simulink model "FOC_Control_doubleLoop"  (R2023a)
settings: Solver=FixedStepDiscrete  StartTime=0.0  StopTime=5  FixedStep=0.000001  RelTol=1e-3  EnableMultiTasking=on
InitFcn:
  | SPEED_PI_P=0.03
  | SPEED_PI_I=5
  | SPEED_PI_UP_LIMIT = 5.0
  | SPEED_PI_LOW_LIMIT = -5.0
  | SPEED_PI_KB = 0.015
  | D_PI_P = 2.199
  | D_PI_I = 1282.8
  | D_PI_UP_LIMIT = 24.0
  | D_PI_LOW_LIMIT = -24.0
  | D_PI_KB = 15
  | Q_PI_P = 2.199
  | Q_PI_I = 1282.8
  | Q_PI_UP_LIMIT = 24.0
  | Q_PI_LOW_LIMIT = -24.0
  | Q_PI_KB = 15
libraries: slpidlib x3, spsDCVoltageSourceLib x1, spsGroundLib x1, spsPermanentMagnetSynchronousMachineLib x1, simulink x1, spsThreePhaseVIMeasurementLib x1, spsUniversalBridgeLib x1, spspowerguiLib x1
settings Model: ExtModeTrigDuration=5  TunableVars=D_PI_I,D_PI_KB,D_PI_LIMIT,D_PI_LOW_LIMIT,D_PI_P,D_PI_UP_LIMIT,Q_PI_I,Q_PI_KB,Q_PI_LIMIT,Q_PI_LOW_LIMIT,Q_PI_P,Q_PI_UP_LIMIT,SPEED_PI_I,SPEED_PI_KB,SPEED_PI_LIMIT,SPEED_PI_LOW_LIMIT,SPEED_PI_P,SPEED_PI_UP_LIMIT  TunableVarsStorageClass=Auto,Auto,Auto,Auto,Auto,Auto,Auto,Auto,Auto,Auto,Auto,Auto,Auto,Auto,Auto,Auto,Auto,Auto  TunableVarsTypeQualifier=,,,,,,,,,,,,,,,,,  Creator=wang  LastModifiedBy=28076
settings SolverCC: AlgebraicLoopSolver=TrustRegion
settings DataIOCC: ReturnWorkspaceOutputs=off
settings OptimizationCC: DefaultParameterBehavior=Inlined  UseDivisionForNetSlopeComputation=on  GainParamInheritBuiltInType=on  UseFloatMulNetSlope=on  DefaultUnderspecifiedDataType=single  InlineInvariantSignals=on  PassReuseOutputArgsAs=Individual arguments  ZeroExternalMemoryAtStartup=off  ZeroInternalMemoryAtStartup=off  NoFixptDivByZeroProtection=on  EfficientFloat2IntCast=on  LifeSpan=1  MaxStackSize=64  OptimizeBlockOrder=speed  DifferentSizesBufferReuse=on  EfficientTunableParamExpr=on
settings DebuggingCC: ParameterTunabilityLossMsg=error  UnconnectedInputMsg=warning  UnconnectedOutputMsg=warning  UnconnectedLineMsg=warning  ArithmeticOperatorsInVariantConditions=warning
settings HardwareCC: ProdBitPerPointer=32  ProdBitPerSizeT=32  ProdBitPerPtrDiffT=32  ProdLargestAtomicInteger=Long  ProdLargestAtomicFloat=Double  ProdWordSize=32  ProdLongLongMode=on  ProdHWDeviceType=ARM Compatible->ARM Cortex
settings ModelReferenceCC: EnableRefExpFcnMdlSchedulingChecks=on
settings SFSimCC: MATLABDynamicMemAlloc=off  CustomCodeUndefinedFunction=UseInterfaceOnly
settings RTWCC: Description=Embedded Coder  SystemTargetFile=ert.tlc  HardwareBoard=NXP FRDM-K64F  TLCOptions="-aInlineSetEventsForThisBaseRateFcn=TLC_FALSE -aSuppressMultiTaskScheduler=TLC_FALSE    -aRateBasedStepFcn=0"  TemplateMakefile=ert_default_tmf  GenerateReport=on  Toolchain=GNU Tools for ARM Embedded Processors  IncludeHyperlinkInReport=on  LaunchReport=on  GenerateTraceInfo=on  GenerateTraceReport=on  GenerateTraceReportSl=on  GenerateTraceReportSf=on  GenerateTraceReportEml=on  GenerateCodeMetricsReport=on  DLArmComputeVersion=19.05
settings CodeAppCC: ForceParamTrailComments=on  IgnoreCustomStorageClasses=off  OperatorAnnotations=on  SimulinkDataObjDesc=on  SFDataObjDesc=on  CustomSymbolStrGlobalVar=rt$N$M  CustomSymbolStrType=$N$M  CustomSymbolStrFcn=$N$M$F  CustomSymbolStrMacro=$N$M  InsertBlockDesc=on
settings ERTTargetCC: CodeReplacementLibrary=ARM Cortex-M (Optimized)  IncludeMdlTerminateFcn=off  CombineSignalStateStructs=on  SupportComplex=off  SupportNonInlinedSFcns=on  ExtModeTransport=4  ExtModeMexFile=sendToCommService  InlinedParameterPlacement=NonHierarchical  ERTSrcFileBannerTemplate=mbd_s32k3_ert_code_template.cgt  ERTHdrFileBannerTemplate=mbd_s32k3_ert_code_template.cgt  ERTDataSrcFileTemplate=mbd_s32k3_ert_code_template.cgt  ERTDataHdrFileTemplate=mbd_s32k3_ert_code_template.cgt  ERTFilePackagingFormat=CompactWithDataFile
settings ConfigComp: PSAutoStubLUT=on

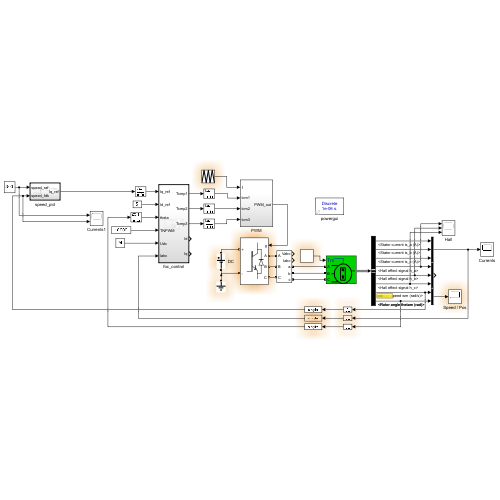
[thumbnail: Simulink's stored preview of the top-level diagram]
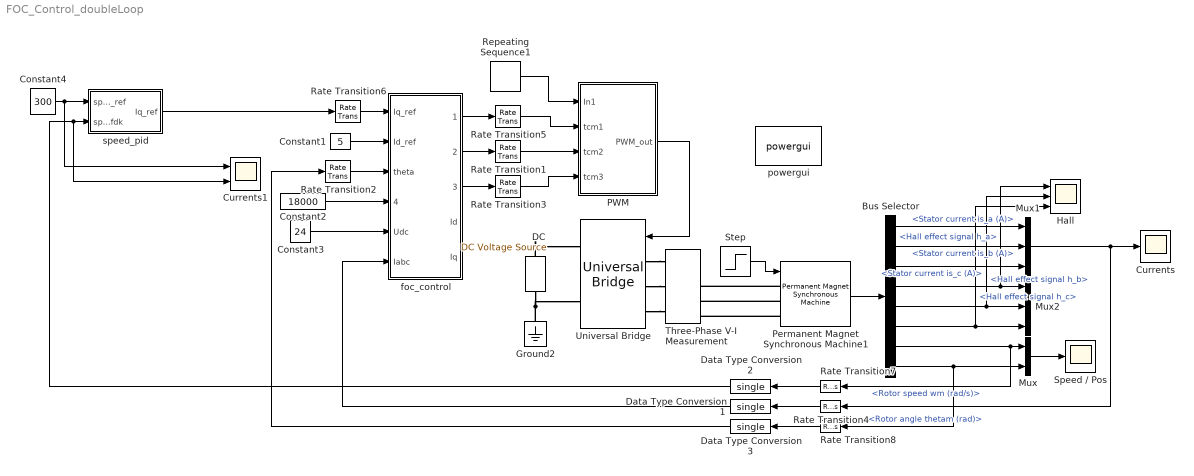
== system FOC_Control_doubleLoop ==
  Bus Selector : BusSelector  OutputSignals=Stator current is_a (A),Stator current is_b (A),Stator current is_c (A),Hall effect signal h_a,Hall effect signal h_b,Hall effect signal h_c,Rotor speed wm (rad/s),Rotor angle thetam (rad)
  Constant1 : Constant  Value=5  OutDataTypeStr=single
  Constant2 : Constant  Value=18000  OutDataTypeStr=single
  Constant3 : Constant  Value=24  OutDataTypeStr=single
  Constant4 : Constant  Value=300  OutDataTypeStr=single
  Currents : Scope
  Currents1 : Scope  NumInputPorts=2
  "DC " : spsDCVoltageSourceLib/DC Voltage Source  Amplitude=24  Measurements=None
  Data Type Conversion1 : DataTypeConversion  OutDataTypeStr=single  SaturateOnIntegerOverflow=off  RndMeth=Floor
  Data Type Conversion2 : DataTypeConversion  OutDataTypeStr=single  SaturateOnIntegerOverflow=off  RndMeth=Floor
  Data Type Conversion3 : DataTypeConversion  OutDataTypeStr=single  SaturateOnIntegerOverflow=off  RndMeth=Floor
  Ground2 : spsGroundLib/Ground  LConnTagsString=a
  Hall : Scope  NumInputPorts=3
  Mux : Mux  Inputs=2
  Mux1 : Mux  Inputs=3
  Mux2 : Mux  Inputs=3
  PWM : Subsystem
  Permanent Magnet Synchronous Machine1 : spsPermanentMagnetSynchronousMachineLib/Permanent Magnet Synchronous Machine  NbPhases=3  FluxDistribution=Sinusoidal  RotorType=Round  MechanicalLoad=Torque Tm  PresetModel=No  ShowDetailedParameters=on  MeasurementBus=off  Resistance=0.6  Inductance=8.5e-3  dqInductances=[8.5e-3, 8.5e-3]  La=1.4e-3  MachineConstant=Flux linkage established by magnets (V.s)  Flux=0.034182  VoltageCst=6.1999  TorqueCst=0.051273  Flat=120  Mechanical=[1.1e-5,1e-4,1,0.02]  PolePairs=4  InitialConditions=[0,0, 0,0]  InitialConditions5ph=[0 0 0 0 0 0]  RefAngle=Aligned with phase A axis (original Park)  IterativeDiscreteModel=Trapezoidal non iterative  TsBlock=-1  TsPowergui=0
  Rate Transition{1..8} (8 alike) : RateTransition
  Repeating Sequence1 : simulink/Sources/Repeating Sequence  rep_seq_t=[0 0.0001 0.0002]  rep_seq_y=[0 9000 0]
  Speed / Pos : Scope
  Step : Step  Time=0  After=0  SampleTime=0
  Three-Phase V-I Measurement : spsThreePhaseVIMeasurementLib/Three-Phase V-I Measurement  VoltageMeasurement=phase-to-ground  SetLabelV=off  LabelV=Vabc  Vpu=off  VpuLL=off  CurrentMeasurement=yes  SetLabelI=off  LabelI=Iabc  Ipu=off  Pbase=100e6  Vbase=500e3  OutputType=Complex  PhasorSimulation=off  PSBequivalent=0
  Universal Bridge : spsUniversalBridgeLib/Universal Bridge  Arms=3  SnubberResistance=1e5  SnubberCapacitance=inf  Device=IGBT / Diodes  Ron=1e-3  Lon=0  ForwardVoltages="[  0  0  ]"  ForwardVoltage=0  GTOparameters=[ 10e-6 , 20e-6 ]  IGBTparameters=[ 1e-6 , 2e-6 ]  Measurements=None  Measurements_2=None  converterType=Rectifier
  foc_control : Subsystem  TreatAsAtomicUnit=on  SystemSampleTime=0.0001
  powergui : spspowerguiLib/powergui  Priority=1  SimulationMode=Discrete  SampleTime=0.000001  frequency=60  Iterations=50  frequencyindice=0  Pbase=100e6  ErrMax=1e-4  UnitsV=kV  UnitsW=MW  buscounter=0  FunctionMessages=off  echomessages=off  EnableUseOfTLC=off  CurrentSourceSwitches=off  DisableSnubberDevices=off  DisableRonSwitches=off  DisableVfSwitches=off  DisplayEquations=off  AutomaticDiscreteSolvers=off  SolverType=Tustin/Backward Euler (TBE)  Interpol=off  ExternalGateDelay=off  methode=off  Ts=100  x0status=blocks  SPID=off  SwTol=0  HookPort=off  NonlinearTolerance=1e-4  nMaxIteration=100  ContinueOnMaxIteration=off  RestoreLinks=warning  ResistiveCurrentMeasurement=off  Frange=[0:2:500]  Ylog=off  Xlog=on  ShowGrid=off  save=off  variable=ZData  structure=0  ZoomFFT=off  StartTime=0.0  cycles=1  DisplayStyle=1  fundamental=60  FreqAxis=off  MaxFrequency=1000  frequencyindicesteady=1  RmsSteady=1  display=off
  speed_pid : Subsystem  TreatAsAtomicUnit=on  SystemSampleTime=0.001
  wires:
  Constant1/1 -> foc_control/2(Id_ref)
  Constant2/1 -> foc_control/4(TNPWM)
  Constant3/1 -> foc_control/5(Udc)
  Repeating Sequence1/1 -> PWM/1(In1)
  foc_control/1(Tcmp1) -> Rate Transition5/1
  foc_control/2(Tcmp2) -> Rate Transition1/1
  foc_control/3(Tcmp3) -> Rate Transition3/1
  PWM/1(PWM_out) -> Universal Bridge/1
  Bus Selector/4 -> Hall/1, Mux2/1  "<Hall effect signal h_a>"
  Mux/1 -> Speed / Pos/1
  Bus Selector/2 -> Mux1/2  "<Stator current is_b (A)>"
  Bus Selector/7 -> Rate Transition7/1, Mux/1  "<Rotor speed wm (rad/s)>"
  Bus Selector/5 -> Mux2/2, Hall/2  "<Hall effect signal h_b>"
  Bus Selector/6 -> Mux2/3, Hall/3  "<Hall effect signal h_c>"
  Mux1/1 -> Rate Transition4/1, Currents/1
  Bus Selector/1 -> Mux1/1  "<Stator current is_a (A)>"
  Bus Selector/8 -> Rate Transition8/1, Mux/2  "<Rotor angle thetam (rad)>"
  Bus Selector/3 -> Mux1/3  "<Stator current is_c (A)>"
  Permanent Magnet Synchronous Machine1/1 -> Bus Selector/1
  Rate Transition2/1 -> foc_control/3(theta)
  Rate Transition5/1 -> PWM/2(tcm1)
  Rate Transition1/1 -> PWM/3(tcm2)
  Rate Transition3/1 -> PWM/4(tcm3)
  Step/1 -> Permanent Magnet Synchronous Machine1/1
  Rate Transition4/1 -> Data Type Conversion1/1
  Data Type Conversion1/1 -> foc_control/6(Iabc)
  Constant4/1 -> Currents1/1, speed_pid/1(speed_ref)
  Rate Transition6/1 -> foc_control/1(Iq_ref)
  Rate Transition7/1 -> Data Type Conversion2/1
  Rate Transition8/1 -> Data Type Conversion3/1
  Data Type Conversion2/1 -> Currents1/2, speed_pid/2(speed_fdk)
  Data Type Conversion3/1 -> Rate Transition2/1
  speed_pid/1(Iq_ref) -> Rate Transition6/1
  connections:
  Ground2/LConn1 -- Universal Bridge/RConn2 -- "DC "/LConn1
  Universal Bridge/LConn1 -- Three-Phase V-I Measurement/LConn1
  Universal Bridge/LConn2 -- Three-Phase V-I Measurement/LConn2
  "DC "/RConn1 -- Universal Bridge/RConn1
  Universal Bridge/LConn3 -- Three-Phase V-I Measurement/LConn3
  Permanent Magnet Synchronous Machine1/LConn1 -- Three-Phase V-I Measurement/RConn1
  Permanent Magnet Synchronous Machine1/LConn2 -- Three-Phase V-I Measurement/RConn2
  Permanent Magnet Synchronous Machine1/LConn3 -- Three-Phase V-I Measurement/RConn3

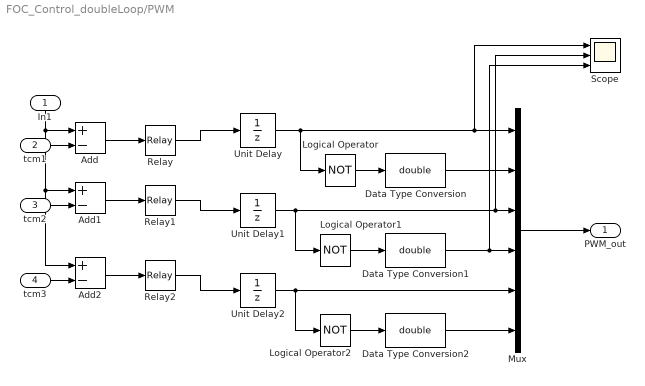
== system FOC_Control_doubleLoop/PWM ==
  In1 : Inport
  tcm1 : Inport  Port=2
  tcm2 : Inport  Port=3
  tcm3 : Inport  Port=4
  Add : Sum  Inputs=+-
  Add1 : Sum  Inputs=+-
  Add2 : Sum  Inputs=+-
  Data Type Conversion : DataTypeConversion  OutDataTypeStr=double  SaturateOnIntegerOverflow=off  RndMeth=Floor
  Data Type Conversion1 : DataTypeConversion  OutDataTypeStr=double  SaturateOnIntegerOverflow=off  RndMeth=Floor
  Data Type Conversion2 : DataTypeConversion  OutDataTypeStr=double  SaturateOnIntegerOverflow=off  RndMeth=Floor
  Logical Operator : Logic  Operator=NOT  AllPortsSameDT=off  OutDataTypeStr=boolean
  Logical Operator1 : Logic  Operator=NOT  AllPortsSameDT=off  OutDataTypeStr=boolean
  Logical Operator2 : Logic  Operator=NOT  AllPortsSameDT=off  OutDataTypeStr=boolean
  Mux : Mux  Inputs=6
  Relay : Relay  OffSwitchValue=-eps
  Relay1 : Relay  OffSwitchValue=-eps
  Relay2 : Relay  OffSwitchValue=-eps
  Scope : Scope  NumInputPorts=3
  Unit Delay : UnitDelay  SampleTime=-1  HasFrameUpgradeWarning=on
  Unit Delay1 : UnitDelay  SampleTime=-1  HasFrameUpgradeWarning=on
  Unit Delay2 : UnitDelay  SampleTime=-1  HasFrameUpgradeWarning=on
  PWM_out : Outport  VectorParamsAs1DForOutWhenUnconnected=off
  wires:
  tcm3/1 -> Add2/2
  tcm2/1 -> Add1/2
  tcm1/1 -> Add/2
  Relay2/1 -> Unit Delay2/1
  Relay1/1 -> Unit Delay1/1
  Relay/1 -> Unit Delay/1
  Unit Delay2/1 -> Mux/5, Logical Operator2/1
  Unit Delay1/1 -> Scope/2, Mux/3, Logical Operator1/1
  Unit Delay/1 -> Logical Operator/1, Scope/1, Mux/1
  Mux/1 -> PWM_out/1
  Data Type Conversion/1 -> Mux/2
  Data Type Conversion1/1 -> Scope/3, Mux/4
  Data Type Conversion2/1 -> Mux/6
  Logical Operator2/1 -> Data Type Conversion2/1
  Logical Operator1/1 -> Data Type Conversion1/1
  Logical Operator/1 -> Data Type Conversion/1
  Add1/1 -> Relay1/1
  Add2/1 -> Relay2/1
  Add/1 -> Relay/1
  In1/1 -> Add/1, Add2/1, Add1/1

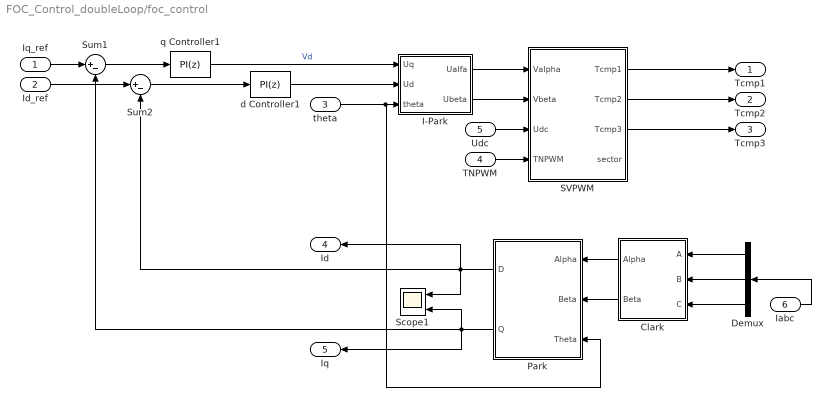
== system FOC_Control_doubleLoop/foc_control ==
  Iq_ref : Inport  OutDataTypeStr=single
  Id_ref : Inport  Port=2  OutDataTypeStr=single
  theta : Inport  Port=3  OutDataTypeStr=single
  TNPWM : Inport  Port=4  OutDataTypeStr=single
  Udc : Inport  Port=5  OutDataTypeStr=single
  Iabc : Inport  Port=6  OutDataTypeStr=single
  Clark : Subsystem
  Demux : Demux  Outputs=3
  I-Park : Subsystem
  Park : Subsystem
  SVPWM : MATLAB Function  TreatAsAtomicUnit=on
  Scope1 : Scope  NumInputPorts=2
  Sum1 : Sum  Inputs=|+-
  Sum2 : Sum  Inputs=|+-
  d Controller1 : slpidlib/PID Controller  Controller=PI  Form=Parallel  TimeDomain=Discrete-time  UseExternalTs=off  SampleTime=-1  IntegratorMethod=Forward Euler  FilterMethod=Forward Euler  ControllerParametersSource=internal  P=D_PI_P  I=D_PI_I  UseKiTs=off  D=0.09  N=100  UseFilter=on  TunerSelectOption=Transfer Function Based (PID Tuner App)  InitialConditionSource=internal  InitialConditionForIntegrator=0  InitialConditionForFilter=0  DifferentiatorICPrevScaledInput=0  ExternalReset=none  TrackingMode=off  Kt=1  LimitOutput=on  SatLimitsSource=internal  UpperSaturationLimit=D_PI_UP_LIMIT  LowerSaturationLimit=D_PI_LOW_LIMIT  LinearizeAsGain=off  AntiWindupMode=back-calculation  Kb=D_PI_KB  LimitIntegrator=off  UpperIntegratorSaturationLimit=inf  LowerIntegratorSaturationLimit=-inf  PGainOutDataTypeStr=single  PProdOutDataTypeStr=single  POutMin=[]  POutMax=[]  IGainOutDataTypeStr=single  IProdOutDataTypeStr=single  IOutMin=[]  IOutMax=[]  DOutMin=[]  DOutMax=[]  NOutMin=[]  NOutMax=[]  SumOutDataTypeStr=single  SumOutMin=[]  SumOutMax=[]  SaturationOutDataTypeStr=single  SaturationOutMin=[]  SaturationOutMax=[]  PParamDataTypeStr=single  PParamMin=[]  PParamMax=[]  IParamDataTypeStr=single  IParamMin=[]  IParamMax=[]  DParamMin=[]  DParamMax=[]  NParamMin=[]  NParamMax=[]  KbParamDataTypeStr=single  KbParamMin=[]  KbParamMax=[]  KtParamMin=[]  KtParamMax=[]  KbOutDataTypeStr=single  KbOutMin=[]  KbOutMax=[]  KtOutMin=[]  KtOutMax=[]  IntegratorOutDataTypeStr=single  IntegratorOutMin=[]  IntegratorOutMax=[]  FilterOutMin=[]  FilterOutMax=[]  SumI1OutDataTypeStr=single  SumI1OutMin=[]  SumI1OutMax=[]  SumI2OutDataTypeStr=single  SumI2OutMin=[]  SumI2OutMax=[]  SumI3OutMin=[]  SumI3OutMax=[]  SumI4OutMin=[]  SumI4OutMax=[]  SumDOutMin=[]  SumDOutMax=[]  SumAccumDataTypeStr=single  SumI1AccumDataTypeStr=single  SumI2AccumDataTypeStr=single  DifferentiatorOutMin=[]  DifferentiatorOutMax=[]  FilterDiffOutCoefMin=[]  FilterDiffOutCoefMax=[]  ReciprocalOutMin=[]  ReciprocalOutMax=[]  SumDenOutMin=[]  SumDenOutMax=[]  SumNumOutMin=[]  SumNumOutMax=[]  DivideOutMin=[]  DivideOutMax=[]  UdiffTsProdOutMin=[]  UdiffTsProdOutMax=[]  NTsProdOutMin=[]  NTsProdOutMax=[]  UintegralTsProdOutMin=[]  UintegralTsProdOutMax=[]  UngainTsProdOutMin=[]  UngainTsProdOutMax=[]  ClampingZeroOutDataTypeStr=Inherit: Inherit via back propagation  ClampingZeroOutMin=[]  ClampingZeroOutMax=[]  FilterDenConstantOutDataTypeStr=Inherit: Inherit via back propagation  FilterDenConstantOutMin=[]  FilterDenConstantOutMax=[]  PCopyOutDataTypeStr=Inherit: Inherit via back propagation  PCopyOutMin=[]  PCopyOutMax=[]  NCopyOutDataTypeStr=Inherit: Inherit via back propagation  NCopyOutMin=[]  NCopyOutMax=[]  IntegratorContinuousStateAttributes=''  IntegratorStateIdentifier=di  IntegratorStateMustResolveToSignalObject=off  IntegratorRTWStateStorageClass=Auto  FilterContinuousStateAttributes=''  FilterStateMustResolveToSignalObject=off  FilterRTWStateStorageClass=Auto  ParallelPVariant=InternalParameters  IdealPVariant=Disabled  IVariant=InternalParameters  DVariant=Disabled  IntegratorVariant=Discrete  SatVariant=Enabled  AWVariant=BackCalculation  PCopyVariant=Disabled  TRVariant=Disabled  FdbkBlocksVariant=Forward  IdealPFdbkVariant=Disabled  SatFdbkVariant=Disabled  DerivativeFilterVariant=Disabled  NVariant=Disabled  NCopyVariant=Disabled_SignalSpec  FilterICVariant=Disabled  IntegratorICVariant=InternalICs  ExternalResetVariant=Disabled  TRSumVariant=Passthrough  SumFdbkVariant=Disabled  SumVariant=Sum_PI  TsampFilterVariant=InternalTs  TsampNgainVariant=Passthrough  TsampIntegralVariant=Disabled_SignalSpec  ExternalSaturationOutDataTypeStr=Inherit: Same as second input
  q Controller1 : slpidlib/PID Controller  Controller=PI  Form=Parallel  TimeDomain=Discrete-time  UseExternalTs=off  SampleTime=-1  IntegratorMethod=Forward Euler  FilterMethod=Forward Euler  ControllerParametersSource=internal  P=Q_PI_P  I=Q_PI_I  UseKiTs=off  D=0.09  N=100  UseFilter=on  TunerSelectOption=Transfer Function Based (PID Tuner App)  InitialConditionSource=internal  InitialConditionForIntegrator=0  InitialConditionForFilter=0  DifferentiatorICPrevScaledInput=0  ExternalReset=none  TrackingMode=off  Kt=1  LimitOutput=on  SatLimitsSource=internal  UpperSaturationLimit=Q_PI_UP_LIMIT  LowerSaturationLimit=Q_PI_LOW_LIMIT  LinearizeAsGain=off  AntiWindupMode=back-calculation  Kb=Q_PI_KB  LimitIntegrator=off  UpperIntegratorSaturationLimit=inf  LowerIntegratorSaturationLimit=-inf  PGainOutDataTypeStr=single  PProdOutDataTypeStr=single  POutMin=[]  POutMax=[]  IGainOutDataTypeStr=single  IProdOutDataTypeStr=single  IOutMin=[]  IOutMax=[]  DOutMin=[]  DOutMax=[]  NOutMin=[]  NOutMax=[]  SumOutDataTypeStr=single  SumOutMin=[]  SumOutMax=[]  SaturationOutDataTypeStr=single  SaturationOutMin=[]  SaturationOutMax=[]  PParamDataTypeStr=single  PParamMin=[]  PParamMax=[]  IParamDataTypeStr=single  IParamMin=[]  IParamMax=[]  DParamMin=[]  DParamMax=[]  NParamMin=[]  NParamMax=[]  KbParamDataTypeStr=single  KbParamMin=[]  KbParamMax=[]  KtParamMin=[]  KtParamMax=[]  KbOutDataTypeStr=single  KbOutMin=[]  KbOutMax=[]  KtOutMin=[]  KtOutMax=[]  IntegratorOutDataTypeStr=single  IntegratorOutMin=[]  IntegratorOutMax=[]  FilterOutMin=[]  FilterOutMax=[]  SumI1OutDataTypeStr=single  SumI1OutMin=[]  SumI1OutMax=[]  SumI2OutDataTypeStr=single  SumI2OutMin=[]  SumI2OutMax=[]  SumI3OutMin=[]  SumI3OutMax=[]  SumI4OutMin=[]  SumI4OutMax=[]  SumDOutMin=[]  SumDOutMax=[]  SumAccumDataTypeStr=single  SumI1AccumDataTypeStr=single  SumI2AccumDataTypeStr=single  DifferentiatorOutMin=[]  DifferentiatorOutMax=[]  FilterDiffOutCoefMin=[]  FilterDiffOutCoefMax=[]  ReciprocalOutMin=[]  ReciprocalOutMax=[]  SumDenOutMin=[]  SumDenOutMax=[]  SumNumOutMin=[]  SumNumOutMax=[]  DivideOutMin=[]  DivideOutMax=[]  UdiffTsProdOutMin=[]  UdiffTsProdOutMax=[]  NTsProdOutMin=[]  NTsProdOutMax=[]  UintegralTsProdOutMin=[]  UintegralTsProdOutMax=[]  UngainTsProdOutMin=[]  UngainTsProdOutMax=[]  ClampingZeroOutDataTypeStr=Inherit: Inherit via back propagation  ClampingZeroOutMin=[]  ClampingZeroOutMax=[]  FilterDenConstantOutDataTypeStr=Inherit: Inherit via back propagation  FilterDenConstantOutMin=[]  FilterDenConstantOutMax=[]  PCopyOutDataTypeStr=Inherit: Inherit via back propagation  PCopyOutMin=[]  PCopyOutMax=[]  NCopyOutDataTypeStr=Inherit: Inherit via back propagation  NCopyOutMin=[]  NCopyOutMax=[]  IntegratorContinuousStateAttributes=''  IntegratorStateIdentifier=qi  IntegratorStateMustResolveToSignalObject=off  IntegratorRTWStateStorageClass=Auto  FilterContinuousStateAttributes=''  FilterStateMustResolveToSignalObject=off  FilterRTWStateStorageClass=Auto  ParallelPVariant=InternalParameters  IdealPVariant=Disabled  IVariant=InternalParameters  DVariant=Disabled  IntegratorVariant=Discrete  SatVariant=Enabled  AWVariant=BackCalculation  PCopyVariant=Disabled  TRVariant=Disabled  FdbkBlocksVariant=Forward  IdealPFdbkVariant=Disabled  SatFdbkVariant=Disabled  DerivativeFilterVariant=Disabled  NVariant=Disabled  NCopyVariant=Disabled_SignalSpec  FilterICVariant=Disabled  IntegratorICVariant=InternalICs  ExternalResetVariant=Disabled  TRSumVariant=Passthrough  SumFdbkVariant=Disabled  SumVariant=Sum_PI  TsampFilterVariant=InternalTs  TsampNgainVariant=Passthrough  TsampIntegralVariant=Disabled_SignalSpec  ExternalSaturationOutDataTypeStr=Inherit: Same as second input
  Tcmp1 : Outport  VectorParamsAs1DForOutWhenUnconnected=off
  Tcmp2 : Outport  Port=2  VectorParamsAs1DForOutWhenUnconnected=off
  Tcmp3 : Outport  Port=3  VectorParamsAs1DForOutWhenUnconnected=off
  Id : Outport  Port=4  VectorParamsAs1DForOutWhenUnconnected=off
  Iq : Outport  Port=5  VectorParamsAs1DForOutWhenUnconnected=off
  wires:
  I-Park/1(Ualfa) -> SVPWM/1(Valpha)
  theta/1 -> Park/3(Theta), I-Park/3(theta)
  I-Park/2(Ubeta) -> SVPWM/2(Vbeta)
  d Controller1/1 -> I-Park/2(Ud)
  Udc/1 -> SVPWM/3(Udc)
  TNPWM/1 -> SVPWM/4(TNPWM)
  SVPWM/1(Tcmp1) -> Tcmp1/1
  SVPWM/2(Tcmp2) -> Tcmp2/1
  SVPWM/3(Tcmp3) -> Tcmp3/1
  Clark/1(Alpha) -> Park/1(Alpha)
  Clark/2(Beta) -> Park/2(Beta)
  Demux/3 -> Clark/3(C)
  Iabc/1 -> Demux/1
  Park/1(D) -> Sum2/2, Id/1, Scope1/1
  Park/2(Q) -> Sum1/2, Iq/1, Scope1/2
  Demux/2 -> Clark/2(B)
  Demux/1 -> Clark/1(A)
  Sum1/1 -> q Controller1/1
  Sum2/1 -> d Controller1/1
  Iq_ref/1 -> Sum1/1
  Id_ref/1 -> Sum2/1
  q Controller1/1 -> I-Park/1(Uq)  "Vd"

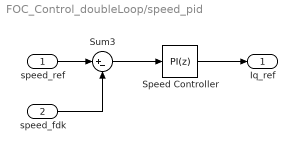
== system FOC_Control_doubleLoop/speed_pid ==
  speed_ref : Inport
  speed_fdk : Inport  Port=2
  Speed Controller : slpidlib/PID Controller  Controller=PI  Form=Ideal  TimeDomain=Discrete-time  UseExternalTs=off  SampleTime=-1  IntegratorMethod=Forward Euler  FilterMethod=Forward Euler  ControllerParametersSource=internal  P=SPEED_PI_P  I=SPEED_PI_I  UseKiTs=off  D=0.0005  N=100  UseFilter=on  TunerSelectOption=Transfer Function Based (PID Tuner App)  InitialConditionSource=internal  InitialConditionForIntegrator=0  InitialConditionForFilter=0  DifferentiatorICPrevScaledInput=0  ExternalReset=none  TrackingMode=off  Kt=1  LimitOutput=on  SatLimitsSource=internal  UpperSaturationLimit=SPEED_PI_UP_LIMIT  LowerSaturationLimit=SPEED_PI_LOW_LIMIT  LinearizeAsGain=off  AntiWindupMode=back-calculation  Kb=SPEED_PI_KB  LimitIntegrator=off  UpperIntegratorSaturationLimit=inf  LowerIntegratorSaturationLimit=-inf  PGainOutDataTypeStr=single  PProdOutDataTypeStr=single  POutMin=[]  POutMax=[]  IGainOutDataTypeStr=single  IProdOutDataTypeStr=single  IOutMin=[]  IOutMax=[]  DOutMin=[]  DOutMax=[]  NOutMin=[]  NOutMax=[]  SumOutDataTypeStr=single  SumOutMin=[]  SumOutMax=[]  SaturationOutDataTypeStr=single  SaturationOutMin=[]  SaturationOutMax=[]  PParamDataTypeStr=single  PParamMin=[]  PParamMax=[]  IParamDataTypeStr=single  IParamMin=[]  IParamMax=[]  DParamMin=[]  DParamMax=[]  NParamMin=[]  NParamMax=[]  KbParamDataTypeStr=single  KbParamMin=[]  KbParamMax=[]  KtParamMin=[]  KtParamMax=[]  KbOutDataTypeStr=single  KbOutMin=[]  KbOutMax=[]  KtOutMin=[]  KtOutMax=[]  IntegratorOutDataTypeStr=single  IntegratorOutMin=[]  IntegratorOutMax=[]  FilterOutMin=[]  FilterOutMax=[]  SumI1OutDataTypeStr=single  SumI1OutMin=[]  SumI1OutMax=[]  SumI2OutDataTypeStr=single  SumI2OutMin=[]  SumI2OutMax=[]  SumI3OutMin=[]  SumI3OutMax=[]  SumI4OutMin=[]  SumI4OutMax=[]  SumDOutMin=[]  SumDOutMax=[]  SumAccumDataTypeStr=single  SumI1AccumDataTypeStr=single  SumI2AccumDataTypeStr=single  DifferentiatorOutMin=[]  DifferentiatorOutMax=[]  FilterDiffOutCoefMin=[]  FilterDiffOutCoefMax=[]  ReciprocalOutMin=[]  ReciprocalOutMax=[]  SumDenOutMin=[]  SumDenOutMax=[]  SumNumOutMin=[]  SumNumOutMax=[]  DivideOutMin=[]  DivideOutMax=[]  UdiffTsProdOutMin=[]  UdiffTsProdOutMax=[]  NTsProdOutMin=[]  NTsProdOutMax=[]  UintegralTsProdOutMin=[]  UintegralTsProdOutMax=[]  UngainTsProdOutMin=[]  UngainTsProdOutMax=[]  ClampingZeroOutDataTypeStr=Inherit: Inherit via back propagation  ClampingZeroOutMin=[]  ClampingZeroOutMax=[]  FilterDenConstantOutDataTypeStr=Inherit: Inherit via back propagation  FilterDenConstantOutMin=[]  FilterDenConstantOutMax=[]  PCopyOutDataTypeStr=Inherit: Inherit via back propagation  PCopyOutMin=[]  PCopyOutMax=[]  NCopyOutDataTypeStr=Inherit: Inherit via back propagation  NCopyOutMin=[]  NCopyOutMax=[]  IntegratorContinuousStateAttributes=''  IntegratorStateIdentifier=si  IntegratorStateMustResolveToSignalObject=off  IntegratorRTWStateStorageClass=Auto  FilterContinuousStateAttributes=''  FilterStateMustResolveToSignalObject=off  FilterRTWStateStorageClass=Auto  ParallelPVariant=Passthrough  IdealPVariant=InternalParameters  IVariant=InternalParameters  DVariant=Disabled  IntegratorVariant=Discrete  SatVariant=Enabled  AWVariant=BackCalculation  PCopyVariant=Disabled  TRVariant=Disabled  FdbkBlocksVariant=Forward  IdealPFdbkVariant=Disabled  SatFdbkVariant=Disabled  DerivativeFilterVariant=Disabled  NVariant=Disabled  NCopyVariant=Disabled_SignalSpec  FilterICVariant=Disabled  IntegratorICVariant=InternalICs  ExternalResetVariant=Disabled  TRSumVariant=Passthrough  SumFdbkVariant=Disabled  SumVariant=Sum_PI  TsampFilterVariant=InternalTs  TsampNgainVariant=Passthrough  TsampIntegralVariant=Disabled_SignalSpec  ExternalSaturationOutDataTypeStr=Inherit: Same as second input
  Sum3 : Sum  Inputs=|+-  InputSameDT=on
  Iq_ref : Outport  VectorParamsAs1DForOutWhenUnconnected=off
  wires:
  Sum3/1 -> Speed Controller/1
  speed_ref/1 -> Sum3/1
  Speed Controller/1 -> Iq_ref/1
  speed_fdk/1 -> Sum3/2

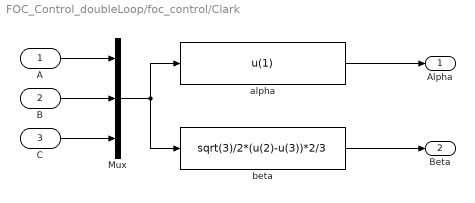
== system FOC_Control_doubleLoop/foc_control/Clark ==
  A : Inport
  B : Inport  Port=2
  C : Inport  Port=3
  Mux : Mux  Inputs=3
  alpha : Fcn  Expr=u(1)
  beta : Fcn  Expr=sqrt(3)/2*(u(2)-u(3))*2/3
  Alpha : Outport  VectorParamsAs1DForOutWhenUnconnected=off
  Beta : Outport  Port=2  VectorParamsAs1DForOutWhenUnconnected=off
  wires:
  alpha/1 -> Alpha/1
  B/1 -> Mux/2
  C/1 -> Mux/3
  A/1 -> Mux/1
  Mux/1 -> beta/1, alpha/1
  beta/1 -> Beta/1

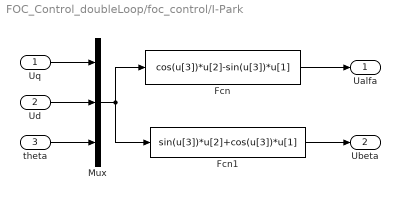
== system FOC_Control_doubleLoop/foc_control/I-Park ==
  Uq : Inport
  Ud : Inport  Port=2
  theta : Inport  Port=3
  Fcn : Fcn  Expr=cos(u[3])*u[2]-sin(u[3])*u[1]
  Fcn1 : Fcn  Expr=sin(u[3])*u[2]+cos(u[3])*u[1]
  Mux : Mux  Inputs=3
  Ualfa : Outport  OutDataTypeStr=single  VectorParamsAs1DForOutWhenUnconnected=off
  Ubeta : Outport  Port=2  OutDataTypeStr=single  VectorParamsAs1DForOutWhenUnconnected=off
  wires:
  Uq/1 -> Mux/1
  Ud/1 -> Mux/2
  theta/1 -> Mux/3
  Mux/1 -> Fcn/1, Fcn1/1
  Fcn/1 -> Ualfa/1
  Fcn1/1 -> Ubeta/1

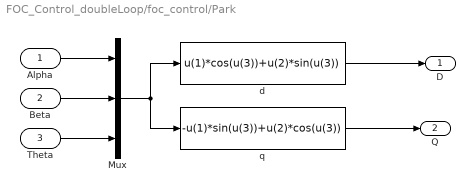
== system FOC_Control_doubleLoop/foc_control/Park ==
  Alpha : Inport
  Beta : Inport  Port=2
  Theta : Inport  Port=3
  Mux : Mux  Inputs=3
  d : Fcn  Expr=u(1)*cos(u(3))+u(2)*sin(u(3))
  q : Fcn  Expr=-u(1)*sin(u(3))+u(2)*cos(u(3))
  D : Outport  VectorParamsAs1DForOutWhenUnconnected=off
  Q : Outport  Port=2  VectorParamsAs1DForOutWhenUnconnected=off
  wires:
  d/1 -> D/1
  Beta/1 -> Mux/2
  Theta/1 -> Mux/3
  Alpha/1 -> Mux/1
  Mux/1 -> q/1, d/1
  q/1 -> Q/1

== matlab function FOC_Control_doubleLoop/foc_control/SVPWM ==
  data: Valpha input single size=1; Tcmp1 output single size=1; Vbeta input single size=1; Tcmp2 output single size=1; Tcmp3 output single size=1; Udc input single size=1; TNPWM input single size=1; sector output single size=1
function [Tcmp1,Tcmp2,Tcmp3,sector] = fcn(Valpha,Vbeta,Udc,TNPWM)
%#codegen

sector = single(0);
Tcmp1 = single(0);
Tcmp2 = single(0);
Tcmp3 = single(0);

%========Parameters statement================

    Vref1 = Vbeta;							                   
    Vref2 = (sqrt(3)*Valpha - Vbeta)/2; 				    
    Vref3 = (-sqrt(3)*Valpha - Vbeta)/2;					
   
 %========Sector calculation=================

  if (Vref1>0)
	   sector = single(1);
  end
  if (Vref2>0)
	   sector = sector+single(2);
  end
  if (Vref3>0)
       sector = sector+single(4);
  end

%======== U1 U2 U3 calculation===================

X = sqrt(3)*Vbeta*TNPWM/Udc;
Y = TNPWM/Udc*(3/2*Valpha+sqrt(3)/2*Vbeta);
Z = TNPWM/Udc*(-3/2*Valpha+sqrt(3)/2*Vbeta);	         

%==========Duty ratio calculation================
switch (sector)   
    case 1
        T1 = Z; T2 = Y; 
	case 2
        T1 = Y; T2 = -X; 
	case 3
        T1 = -Z; T2 = X; 
	case 4
        T1 = -X; T2 = Z;
	case 5
        T1 = X; T2 = -Y;
    otherwise
        T1 = -Y; T2 = -Z;
end

f_temp = (T1+T2);
if f_temp > TNPWM
    T1 = T1/f_temp*TNPWM;
    T2 = T2/f_temp*TNPWM;
else
    T1 = T1;
    T2 = T2;
end

ta = (TNPWM-(T1+T2))/4.0;
tb = ta+T1/2;
tc = tb+T2/2;

%==========Duty ratio calculation================
switch (sector)
    case 1 
        Tcmp1=tb;
        Tcmp2=ta;
        Tcmp3=tc; 
        
    case 2 
        Tcmp1=ta;
        Tcmp2=tc;
        Tcmp3=tb; 
       
    case 3 
        Tcmp1=ta;
        Tcmp2=tb;
        Tcmp3=tc; 
        
    case 4 
        Tcmp1=tc;
        Tcmp2=tb;
        Tcmp3=ta;
        
    case 5 
        Tcmp1=tc;
        Tcmp2=ta;
        Tcmp3=tb;
        
   case 6
       Tcmp1=tb;
       Tcmp2=tc;
       Tcmp3=ta;
end
end
